simulink model "hw5_4"  (R2023a)
settings: Solver=VariableStepAuto  StartTime=0.0  StopTime=10.0  RelTol=1e-3
libraries: simulink x1
settings Model: Creator=마이컴  LastModifiedBy=마이컴

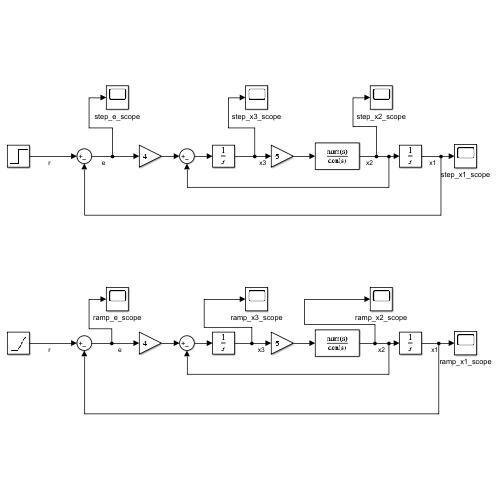
[thumbnail: Simulink's stored preview of the top-level diagram]
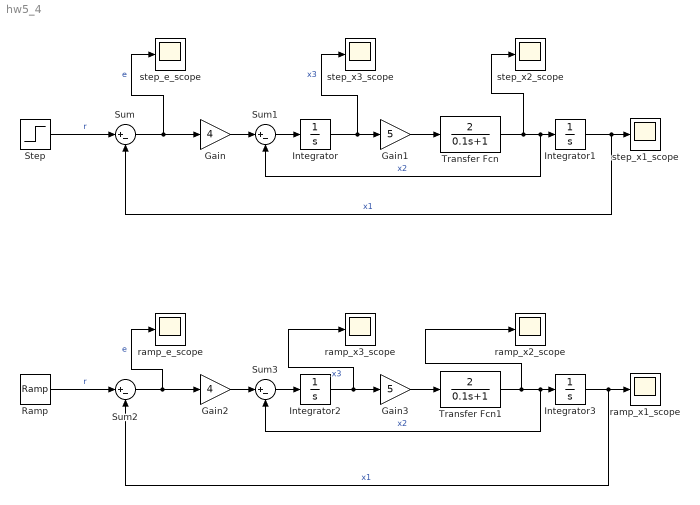
== system hw5_4 ==
  Gain : Gain  Gain=4
  Gain1 : Gain  Gain=5
  Gain2 : Gain  Gain=4
  Gain3 : Gain  Gain=5
  Integrator{,1..3} (4 alike) : Integrator
  Ramp : simulink/Sources/Ramp  slope=1  start=0  InitialOutput=0
  Step : Step  SampleTime=0
  Sum{,1..3} (4 alike) : Sum  Inputs=|+-
  Transfer Fcn : TransferFcn  Numerator=[2]  Denominator=[0.1 1]
  Transfer Fcn1 : TransferFcn  Numerator=[2]  Denominator=[0.1 1]
  ramp_e_scope : Scope
  ramp_x1_scope : Scope
  ramp_x2_scope : Scope
  ramp_x3_scope : Scope
  step_e_scope : Scope
  step_x1_scope : Scope
  step_x2_scope : Scope
  step_x3_scope : Scope
  wires:
  Integrator/1 -> step_x3_scope/1, Gain1/1  "x3"
  Sum1/1 -> Integrator/1
  Gain/1 -> Sum1/1
  Sum/1 -> step_e_scope/1, Gain/1  "e"
  Gain1/1 -> Transfer Fcn/1
  Transfer Fcn/1 -> step_x2_scope/1, Sum1/2, Integrator1/1  "x2"
  Integrator1/1 -> step_x1_scope/1, Sum/2  "x1"
  Step/1 -> Sum/1  "r"
  Ramp/1 -> Sum2/1  "r"
  Integrator3/1 -> ramp_x1_scope/1, Sum2/2  "x1"
  Transfer Fcn1/1 -> ramp_x2_scope/1, Integrator3/1, Sum3/2  "x2"
  Gain3/1 -> Transfer Fcn1/1
  Sum2/1 -> ramp_e_scope/1, Gain2/1  "e"
  Gain2/1 -> Sum3/1
  Sum3/1 -> Integrator2/1
  Integrator2/1 -> ramp_x3_scope/1, Gain3/1  "x3"
